simulink model "Friction_04_Disk_Rolling_on_Ramp"  (R2014b)
settings: Solver=ode15s  StartTime=0.0  StopTime=4  MaxStep=1e-2  RelTol=1e-4  AbsTol=1e-5
PostLoadFcn:
  | warning off Simulink:Engine:UsingDefaultMaxStepSize
StartFcn:
  | tic;
StopFcn:
  | Elapsed_Sim_Time = toc;
  | disp(['Elapsed Sim Time = ' num2str(Elapsed_Sim_Time)]);
undefined symbols (not defined in the file): X, Y, Z
libraries: sm_lib x9, nesl_utility x3, Contact_Forces_Lib x1, Parts_Lib x1, simulink x1
Description:
  | Copyright 2015 The MathWorks, Inc.
settings Model: Creator=smiller  LastModifiedBy=smiller
settings DataIOCC: LimitDataPoints=off  SignalLoggingSaveFormat=ModelDataLogs
settings OptimizationCC: ExpressionDepthLimit=2147483647
settings DebuggingCC: UnderspecifiedInitializationDetection=Classic  MergeDetectMultiDrivingBlocksExec=none  IgnoredZcDiagnostic=none  FcnCallInpInsideContextMsg=EnableAllAsWarning  FrameProcessingCompatibilityMsg=error  StateNameClashWarn=warning
settings SimscapeCC: SimscapeLogType=all  SimscapeLogLimitData=off
settings DiagnosticsConfigSet: SimMechanicsRigidlyBoundBlock=none
settings ExplorerConfigSet: InternalSimMechanicsExplorerSettings="<ExplorerConfiguration><canonicalview>default</canonicalview><AnimationSetting><BasePlaybackSpeed>1.0</BasePlaybackSpeed><PlaybackSpeedFactor>1.0</PlaybackSpeedFactor></AnimationSetting><TilePanel><TileInfo><Tiles Columns=\"1\" Count=\"1\" Rows=\"1\"><Column Left=\"2\" Weight=\"1\"/><Column Left=\"676\"/><Row Top=\"2\" Weight=\"1\"/><Row Top=\"798\"/><Tile Height=\"1\" Width=\"1\" X=\"0\" Y=\"0\"/></Tiles></TileInfo><SceneInfo><SceneViewer><BGColor><R>0.91372549533843994</R><G>0.9529411792755127</G><B>0.9529411792755127</B></BGColor><Camera><Position><X>0.2122427225112915</X><Y>-3.2228425197050803</Y><Z>0.071312487125396729</Z></Position><Center><X>0.2122427225112915</X><Y>0</Y><Z>0.071312487125396729</Z></Center><Up><X>0</X><Y>-0</Y><Z>1</Z></Up><Left>-1.5199732482433319</Left><Right>1.5199732482433319</Right><Bottom>-0.32864254564046863</Bottom><Top>0.32864254564046863</Top></Camera></SceneViewer></SceneInfo></TilePanel></ExplorerConfiguration>"

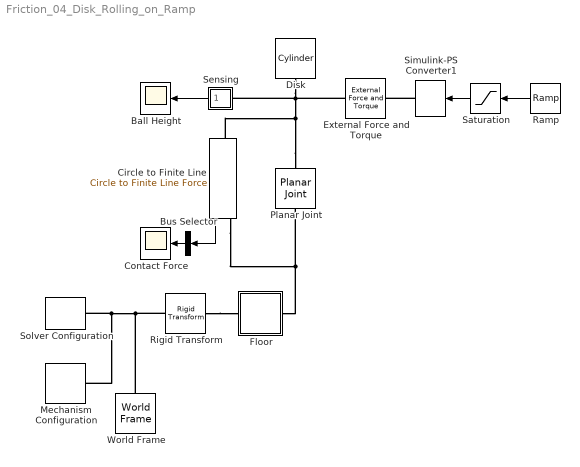
== system Friction_04_Disk_Rolling_on_Ramp ==
  Ball Height : Scope
      settings: TimeRange=10  YMin=-0.9962222222222152  YMax=2.527037037037044
  Bus Selector : BusSelector  OutputSignals=Normal Force  OutputAsBus=on
  Circle to Finite Line : Contact_Forces_Lib/2D/Circle to Finite Line Force  circle_rad=0.2  line_depth=0.05/2  line_length=0.5*5  force_law=Linear  k_contact=1e5  b_contact=1e3  pen_full_damp_F=1e-4  pen_exponent=1  custom_param_1=1  custom_param_2=1  friction_law=Stick-Slip Continuous  mu_kinetic=0.5  mu_static=0.7  v_thr=0.001
  Contact Force : Scope
      settings: YMin=0  YMax=2000
  Disk : Parts_Lib/Cylinder  cyl_radius=0.2  cyl_length=0.2  cyl_density=1000  cyl_color=red  cyl_opacity=1  mark_radius=[0.75 0.5]  mark_angle=60  mark_color=purple  mark_opacity=1
  External Force and Torque : sm_lib/Forces and Torques/External Force and Torque  ForceResolutionFrame=AttachedFrame  EnableForceX=off  EnableForceY=off  EnableForceZ=off  EnableForce=off  TorqueResolutionFrame=AttachedFrame  EnableTorqueX=off  EnableTorqueY=off  EnableTorqueZ=on  EnableTorque=off  BlockFunction=simmechanics.library.forces_torques.external_force_torque
  Floor : Subsystem
  Mechanism Configuration : sm_lib/Utilities/Mechanism Configuration  UniformGravity=Constant  GravityVector=[0 0 -9.81]  GravityUnits=m/s^2  LinearizationDelta=0.001  BlockFunction=simmechanics.library.utilities.mechanism_configuration
  Planar Joint : sm_lib/Joints/Planar Joint  SenseConstraintForce=off  SenseConstraintForceX=off  SenseConstraintForceY=off  SenseConstraintForceZ=off  SenseConstraintTorque=off  SenseConstraintTorqueX=off  SenseConstraintTorqueY=off  SenseConstraintTorqueZ=off  SenseTotalForce=off  SenseTotalForceX=off  SenseTotalForceY=off  SenseTotalForceZ=off  SenseTotalTorque=off  SenseTotalTorqueX=off  SenseTotalTorqueY=off  SenseTotalTorqueZ=off  CompositeWrenchDir=FollowerOnBase  CompositeWrenchFrame=BaseFrame  PxEquilibriumPosition=0  PxEquilibriumPositionUnits=m  PxSpringStiffness=0  PxSpringStiffnessUnits=N/m  PxDampingCoefficient=0  PxDampingCoefficientUnits=N/(m/s)  PxTorqueActuationMode=NoTorque  PxMotionActuationMode=ComputedMotion  PxSensePosition=off  PxSenseVelocity=off  PxSenseAcceleration=off  PxSenseTorqueForce=off  PxPositionTargetValue=0.5  PxPositionTargetValueUnits=m  PxPositionTargetSpecify=on  PxPositionTargetPriority=High  PxVelocityTargetValue=0  PxVelocityTargetValueUnits=m/s  PxVelocityTargetSpecify=off  PxVelocityTargetPriority=High  PyEquilibriumPosition=0  PyEquilibriumPositionUnits=m  PySpringStiffness=0  PySpringStiffnessUnits=N/m  PyDampingCoefficient=0  PyDampingCoefficientUnits=N/(m/s)  PyTorqueActuationMode=NoTorque  PyMotionActuationMode=ComputedMotion  PySensePosition=off  PySenseVelocity=off  PySenseAcceleration=off  PySenseTorqueForce=off  PyPositionTargetValue=0.8  PyPositionTargetValueUnits=m  PyPositionTargetSpecify=on  PyPositionTargetPriority=High  PyVelocityTargetValue=-0.2*0  PyVelocityTargetValueUnits=m/s  PyVelocityTargetSpecify=off  PyVelocityTargetPriority=High  RzEquilibriumPosition=0  RzEquilibriumPositionUnits=deg  RzSpringStiffness=0  RzSpringStiffnessUnits=N*m/deg  RzDampingCoefficient=0  RzDampingCoefficientUnits=N*m/(deg/s)  RzTorqueActuationMode=NoTorque  RzMotionActuationMode=ComputedMotion  RzSensePosition=off  RzSenseVelocity=off  RzSenseAcceleration=off  RzSenseTorqueForce=off  RzPositionTargetValue=0  RzPositionTargetValueUnits=deg  RzPositionTargetSpecify=off  RzPositionTargetPriority=High  RzVelocityTargetValue=10*0  RzVelocityTargetValueUnits=rad/s  RzVelocityTargetSpecify=on  RzVelocityTargetPriority=High  BlockFunction=simmechanics.library.joints.planar_joint
  Ramp : simulink/Sources/Ramp  slope=30  start=1  X0=0
  Rigid Transform : sm_lib/Frames and Transforms/Rigid Transform  TranslationMethod=None  TranslationLengthUnit=m  TranslationStandardAxis=+Z  TranslationStandardOffset=0  TranslationCartesianOffset=[0 0 0]  TranslationROffset=0  TranslationROffsetUnits=m  TranslationZOffset=0  TranslationZOffsetUnits=m  TranslationThetaOffset=0  TranslationThetaOffsetUnits=deg  RotationMethod=StandardAxis  RotationAngleUnits=deg  RotationStandardAxis=+Y  RotationAngle=-10  RotationArbitraryAxis=[0 0 1]  FollAlignAxisA=+X  BaseAlignAxisA=+Y  FollAlignAxisB=+Y  BaseAlignAxisB=+Z  RotationMatrix=[1 0 0; 0 1 0; 0 0 1]  BlockFunction=simmechanics.library.frames_transforms.rigid_transform
  Saturation : Saturate  UpperLimit=25  LowerLimit=-25
  Sensing : Subsystem
      mask Display: disp('S')
  Simulink-PS Converter1 : nesl_utility/Simulink-PS Converter  PhysicalDomain=network_engine_domain  SubClassName=ps_input  LeftPortType=input  RightPortType=output  PseudoPeriodic=off  Frequencies=[]  NoiseDistribution=none  NoiseParameters=[]  Unit=1  AffineConversion=off  InputFiltering=off  SimscapeFilterOrder=1  InputFilterTimeConstant=0.001  UdotUserProvided=1
  Solver Configuration : nesl_utility/Solver Configuration  PhysicalDomain=network_engine_domain  SubClassName=solver  LeftPortType=input  RightPortType=generic  Accelerate=off  Tones=[]  Harmonics=[]  SimulateNoise=off  Profile=off  UseLocalSampling=off  EnableSwitchedLinearOptims=on  FrequencyDomain=off  UseCCode=off  RelTol=0.001  AbsTol=1e-06  MinStep=1e-09  ToWorkspace=off  DoDC=off  ResidualTolerance=1e-9  UseLocalSolver=off  LocalSolverChoice=NE_BACKWARD_EULER_ADVANCER  LocalSolverSampleTime=.001  DoFixedCost=off  MaxNonlinIter=3  MaxModeIter=2  LinearAlgebra=Sparse  DelaysMemoryBudget=1024  AutomaticFiltering=on  FilteringTimeConstant=0.001
  World Frame : sm_lib/Frames and Transforms/World Frame  BlockFunction=simmechanics.library.frames_transforms.world_frame
  wires:
  Sensing/1(S) -> Ball Height/1
  Circle to Finite Line/1 -> Bus Selector/1
  Bus Selector/1 -> Contact Force/1
  Ramp/1 -> Saturation/1
  Saturation/1 -> Simulink-PS Converter1/1
  connections:
  Planar Joint/RConn1 -- Disk/LConn1 -- External Force and Torque/RConn1 -- Sensing/LConn1 -- Circle to Finite Line/LConn1
  Floor/RConn1 -- Circle to Finite Line/RConn1 -- Planar Joint/LConn1
  World Frame/RConn1 -- Rigid Transform/LConn1 -- Mechanism Configuration/RConn1 -- Solver Configuration/RConn1
  Simulink-PS Converter1/RConn1 -- External Force and Torque/LConn1
  Rigid Transform/RConn1 -- Floor/LConn1

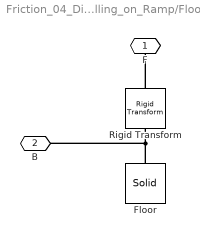
== system Friction_04_Disk_Rolling_on_Ramp/Floor ==
  Floor : sm_lib/Body Elements/Solid  InertiaType=CalculateFromGeometry  Mass=1  MassUnits=kg  CenterOfMass=[0 0 0]  CenterOfMassUnits=m  MomentsOfInertia=[1 1 1]  MomentsOfInertiaUnits=kg*m^2  ProductsOfInertia=[0 0 0]  ProductsOfInertiaUnits=kg*m^2  DensityBased=on  Density=1000  DensityUnits=kg/(m^3)  GraphicType=FromGeometry  MarkerShape=Sphere  MarkerSize=10  MarkerSizeUnits=m  GraphicVisPropType=SimpleVisualProperties  GraphicDiffuseColor=[0.5 0.5 0.5]  GraphicSpecularColor=[0.5 0.5 0.5 1.0]  GraphicAmbientColor=[0.15 0.15 0.15 1.0]  GraphicEmissiveColor=[0.0 0.0 0.0 1.0]  GraphicShininess=75  GraphicOpacity=1.0  GeometryShape=Brick  RectangleSize=[1 1]  RectangleSizeUnits=m  BrickDimensions=[0.5*5 0.2 0.05]  BrickDimensionUnits=m  CylinderRadius=1  CylinderRadiusUnits=m  CylinderLength=1  CylinderLengthUnits=m  SphereRadius=1  SphereRadiusUnits=m  EllipsoidRadii=[1 1 1]  EllipsoidRadiiUnits=m  ExtrusionCrossSection=[1 1; -1 1; -1 -1; 1 -1]  ExtrusionCrossSectionUnits=m  ExtrusionLength=1  ExtrusionLengthUnits=m  PolygonNumSides=3  PolygonOuterRadius=1  PolygonOuterRadiusUnits=m  ExtGeomFileType=STL  ExtGeomFileUnits=m  RevolutionCrossSection=[1 1; 1 -1; 2 -1; 2 1]  RevolutionCrossSectionUnits=m  RevolutionExtent=Full  RevolutionAngle=180  RevolutionAngleUnits=deg  BlockFunction=simmechanics.library.body_elements.solid
  Rigid Transform : sm_lib/Frames and Transforms/Rigid Transform  TranslationMethod=None  TranslationLengthUnit=m  TranslationStandardAxis=+Z  TranslationStandardOffset=0  TranslationCartesianOffset=[0 0 0]  TranslationROffset=0  TranslationROffsetUnits=m  TranslationZOffset=0  TranslationZOffsetUnits=m  TranslationThetaOffset=0  TranslationThetaOffsetUnits=deg  RotationMethod=AlignedAxes  RotationAngleUnits=deg  RotationStandardAxis=+Z  RotationAngle=0  RotationArbitraryAxis=[0 0 1]  FollAlignAxisA=+X  BaseAlignAxisA=+Z  FollAlignAxisB=+Y  BaseAlignAxisB=+X  RotationMatrix=[1 0 0; 0 1 0; 0 0 1]  BlockFunction=simmechanics.library.frames_transforms.rigid_transform
  F : PMIOPort  Port=1  Side=Right
  B : PMIOPort  Port=2  Side=Left
  connections:
  Floor/RConn1 -- B/RConn1 -- Rigid Transform/LConn1
  Rigid Transform/RConn1 -- F/RConn1

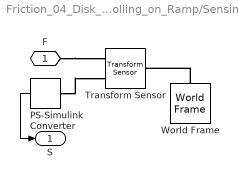
== system Friction_04_Disk_Rolling_on_Ramp/Sensing ==
  PS-Simulink Converter : nesl_utility/PS-Simulink Converter  PhysicalDomain=network_engine_domain  SubClassName=ps_output  LeftPortType=input  RightPortType=output  PseudoPeriodic=off  Frequencies=[]  Unit=1  AffineConversion=off
  Transform Sensor : sm_lib/Frames and Transforms/Transform Sensor  MeasurementFrame=World  SenseAngle=off  SenseAxis=off  SenseAngle1=off  SenseAngle2=off  SenseAngle3=off  SenseQ=off  SenseR=off  SenseOmegaX=off  SenseOmegaY=off  SenseOmegaZ=off  SenseOmega1=off  SenseOmega2=off  SenseOmega3=off  SenseQDot=off  SenseRDot=off  SenseAlphaX=off  SenseAlphaY=off  SenseAlphaZ=off  SenseAlpha1=off  SenseAlpha2=off  SenseAlpha3=off  SenseQDDot=off  SenseRDDot=off  SenseX=off  SenseY=off  SenseZ=on  SenseRad=off  SenseAzim=off  SenseDist=off  SenseInc=off  SenseXDot=off  SenseYDot=off  SenseZDot=off  SenseRadDot=off  SenseAzimDot=off  SenseDistDot=off  SenseIncDot=off  SenseXDDot=off  SenseYDDot=off  SenseZDDot=off  SenseRadDDot=off  SenseAzimDDot=off  SenseDistDDot=off  SenseIncDDot=off  BlockFunction=simmechanics.library.frames_transforms.transform_sensor
  World Frame : sm_lib/Frames and Transforms/World Frame  BlockFunction=simmechanics.library.frames_transforms.world_frame
  F : PMIOPort  Port=1  Side=Left
  S : Outport
  wires:
  PS-Simulink Converter/1 -> S/1
  connections:
  World Frame/RConn1 -- Transform Sensor/LConn1
  F/RConn1 -- Transform Sensor/RConn1
  PS-Simulink Converter/LConn1 -- Transform Sensor/RConn2
